simulink library "csc_pwr_power_system_sim_lib"  (R2014b)
settings: Solver=ode45  SolverMode=SingleTasking  StartTime=0.0  StopTime=10.0  RelTol=1e-3
libraries: util_info_lib x1, csc_swm_switch_state_model_collection_lib x1
settings Model: ExtModeAutoUpdateStatusClock=off  Creator=hcannon  LastModifiedBy=mstewart

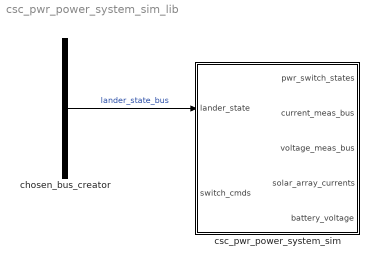
== system csc_pwr_power_system_sim_lib ==
  chosen_bus_creator : BusCreator  Inputs=7  OutDataTypeStr=Bus: lander_state_bus  NonVirtualBus=on
  csc_pwr_power_system_sim : Subsystem
  wires:
  chosen_bus_creator/1 -> csc_pwr_power_system_sim/1(lander_state)  "lander_state_bus"
  ? -> chosen_bus_creator/1  "rrd_alpha_body_in_eci"
  ? -> chosen_bus_creator/2  "rrk_rate_body_eci_body"
  ? -> chosen_bus_creator/3  "rrk_q_body_from_eci"
  ? -> chosen_bus_creator/4  "rrk_euler_zyx_rot_deg"
  ? -> chosen_bus_creator/5  "rtd_acc_body_in_eci"
  ? -> chosen_bus_creator/6  "rtk_vel_eci"
  ? -> chosen_bus_creator/7  "rtk_pos_eci"

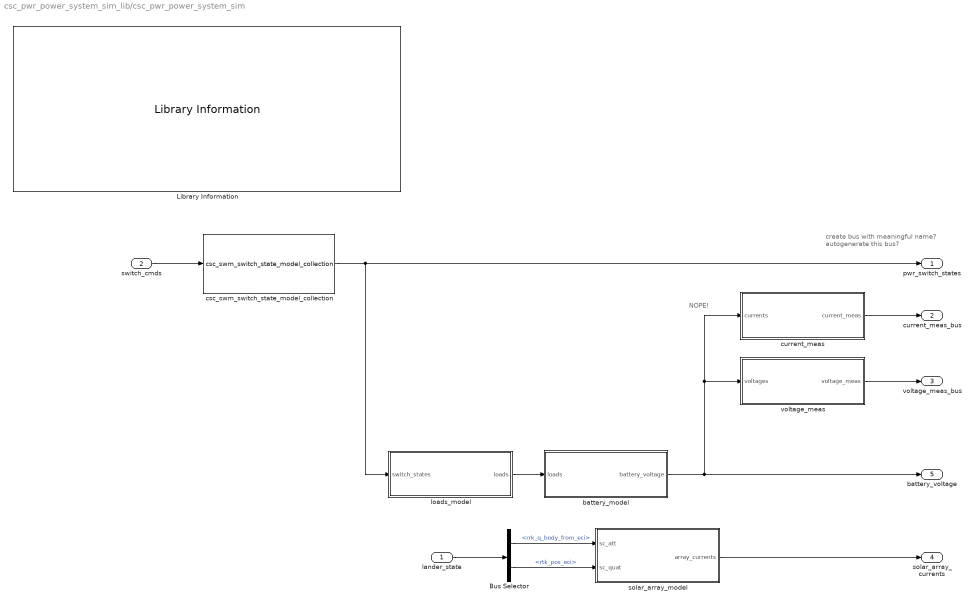
== system csc_pwr_power_system_sim_lib/csc_pwr_power_system_sim ==
  note: create bus with meaningful name?
      | autogenerate this bus?
  note: NOPE!
  lander_state : Inport
  switch_cmds : Inport  Port=2
  Bus Selector : BusSelector  OutputSignals=rrk_q_body_from_eci,rtk_pos_eci
  Library Information : util_info_lib/Library Information  owner='escrane'
  battery_model : Subsystem
  csc_swm_switch_state_model_collection : csc_swm_switch_state_model_collection_lib/csc_swm_switch_state_model_collection  SystemSampleTime=-1
  current_meas : Subsystem
  loads_model : Subsystem
  solar_array_model : Subsystem
  voltage_meas : Subsystem
  pwr_switch_states : Outport
  current_meas_bus : Outport  Port=2
  voltage_meas_bus : Outport  Port=3
  solar_array_currents : Outport  Port=4
  battery_voltage : Outport  Port=5
  wires:
  current_meas/1(current_meas) -> current_meas_bus/1
  voltage_meas/1(voltage_meas) -> voltage_meas_bus/1
  battery_model/1(battery_voltage) -> battery_voltage/1, voltage_meas/1(voltages), current_meas/1(currents)
  solar_array_model/1(array_currents) -> solar_array_currents/1
  switch_cmds/1 -> csc_swm_switch_state_model_collection/1
  loads_model/1(loads) -> battery_model/1(loads)
  csc_swm_switch_state_model_collection/1 -> loads_model/1(switch_states), pwr_switch_states/1
  Bus Selector/1 -> solar_array_model/1(sc_att)  "<rrk_q_body_from_eci>"
  Bus Selector/2 -> solar_array_model/2(sc_quat)  "<rtk_pos_eci>"
  lander_state/1 -> Bus Selector/1

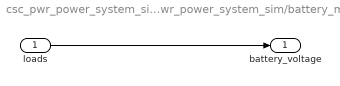
== system csc_pwr_power_system_sim_lib/csc_pwr_power_system_sim/battery_model ==
  loads : Inport
  battery_voltage : Outport
  wires:
  loads/1 -> battery_voltage/1

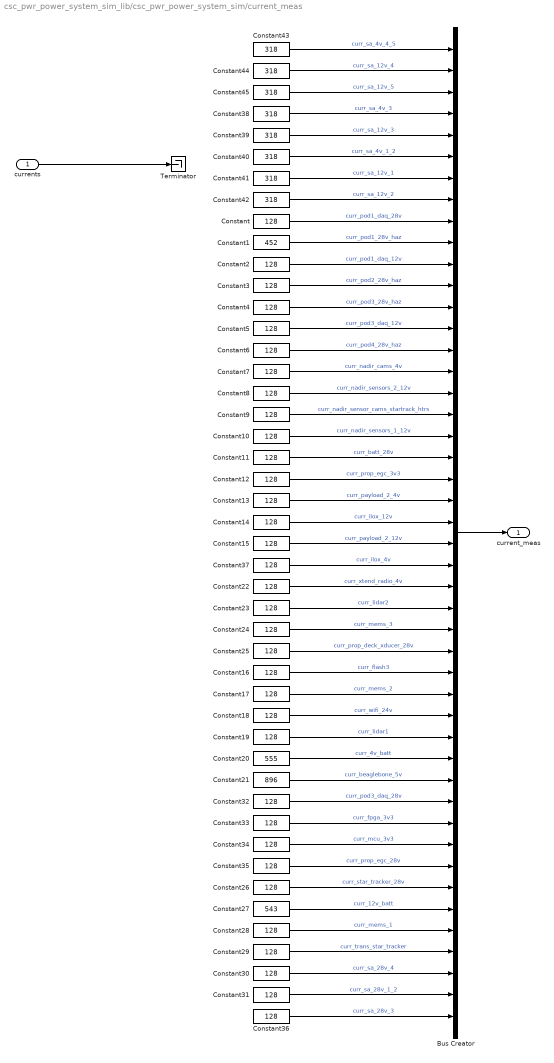
== system csc_pwr_power_system_sim_lib/csc_pwr_power_system_sim/current_meas ==
  currents : Inport
  Bus Creator : BusCreator  Inputs=46
  Constant{,2..19,22..26,28..37} (34 alike) : Constant  Value=128  OutDataTypeStr=uint16
  Constant1 : Constant  Value=452  OutDataTypeStr=uint16
  Constant20 : Constant  Value=555  OutDataTypeStr=uint16
  Constant21 : Constant  Value=896  OutDataTypeStr=uint16
  Constant27 : Constant  Value=543  OutDataTypeStr=uint16
  Constant{38..45} (8 alike) : Constant  Value=318  OutDataTypeStr=uint16
  Terminator : Terminator
  current_meas : Outport
  wires:
  Constant42/1 -> Bus Creator/8  "curr_sa_12v_2"
  Constant41/1 -> Bus Creator/7  "curr_sa_12v_1"
  Constant40/1 -> Bus Creator/6  "curr_sa_4v_1_2"
  Constant39/1 -> Bus Creator/5  "curr_sa_12v_3"
  Constant38/1 -> Bus Creator/4  "curr_sa_4v_3"
  Constant45/1 -> Bus Creator/3  "curr_sa_12v_5"
  Constant44/1 -> Bus Creator/2  "curr_sa_12v_4"
  Constant43/1 -> Bus Creator/1  "curr_sa_4v_4_5"
  Constant36/1 -> Bus Creator/46  "curr_sa_28v_3"
  Constant31/1 -> Bus Creator/45  "curr_sa_28v_1_2"
  Constant30/1 -> Bus Creator/44  "curr_sa_28v_4"
  Constant29/1 -> Bus Creator/43  "curr_trans_star_tracker"
  Constant28/1 -> Bus Creator/42  "curr_mems_1"
  Constant27/1 -> Bus Creator/41  "curr_12v_batt"
  Constant26/1 -> Bus Creator/40  "curr_star_tracker_28v"
  Constant35/1 -> Bus Creator/39  "curr_prop_egc_28v"
  Constant34/1 -> Bus Creator/38  "curr_mcu_3v3"
  Constant33/1 -> Bus Creator/37  "curr_fpga_3v3"
  Constant32/1 -> Bus Creator/36  "curr_pod3_daq_28v"
  Constant21/1 -> Bus Creator/35  "curr_beaglebone_5v"
  Constant20/1 -> Bus Creator/34  "curr_4v_batt"
  Constant19/1 -> Bus Creator/33  "curr_lidar1"
  Constant18/1 -> Bus Creator/32  "curr_wifi_24v"
  Constant17/1 -> Bus Creator/31  "curr_mems_2"
  Constant16/1 -> Bus Creator/30  "curr_flash3"
  Constant25/1 -> Bus Creator/29  "curr_prop_deck_xducer_28v"
  Constant24/1 -> Bus Creator/28  "curr_mems_3"
  Constant23/1 -> Bus Creator/27  "curr_lidar2"
  Constant22/1 -> Bus Creator/26  "curr_xtend_radio_4v"
  Constant37/1 -> Bus Creator/25  "curr_ilox_4v"
  Constant15/1 -> Bus Creator/24  "curr_payload_2_12v"
  Constant14/1 -> Bus Creator/23  "curr_ilox_12v"
  Constant13/1 -> Bus Creator/22  "curr_payload_2_4v"
  Constant12/1 -> Bus Creator/21  "curr_prop_egc_3v3"
  Constant11/1 -> Bus Creator/20  "curr_batt_28v"
  Constant10/1 -> Bus Creator/19  "curr_nadir_sensors_1_12v"
  Constant9/1 -> Bus Creator/18  "curr_nadir_sensor_cams_startrack_htrs"
  Constant8/1 -> Bus Creator/17  "curr_nadir_sensors_2_12v"
  Bus Creator/1 -> current_meas/1
  Constant7/1 -> Bus Creator/16  "curr_nadir_cams_4v"
  Constant6/1 -> Bus Creator/15  "curr_pod4_28v_haz"
  Constant5/1 -> Bus Creator/14  "curr_pod3_daq_12v"
  Constant4/1 -> Bus Creator/13  "curr_pod3_28v_haz"
  Constant3/1 -> Bus Creator/12  "curr_pod2_28v_haz"
  Constant2/1 -> Bus Creator/11  "curr_pod1_daq_12v"
  Constant1/1 -> Bus Creator/10  "curr_pod1_28v_haz"
  Constant/1 -> Bus Creator/9  "curr_pod1_daq_28v"
  currents/1 -> Terminator/1

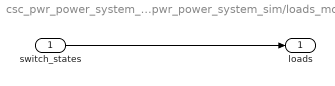
== system csc_pwr_power_system_sim_lib/csc_pwr_power_system_sim/loads_model ==
  switch_states : Inport
  loads : Outport
  wires:
  switch_states/1 -> loads/1

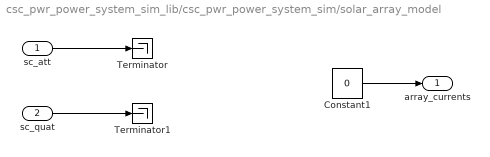
== system csc_pwr_power_system_sim_lib/csc_pwr_power_system_sim/solar_array_model ==
  sc_att : Inport
  sc_quat : Inport  Port=2
  Constant1 : Constant  Value=0  OutDataTypeStr=double
  Terminator : Terminator
  Terminator1 : Terminator
  array_currents : Outport
  wires:
  sc_att/1 -> Terminator/1
  sc_quat/1 -> Terminator1/1
  Constant1/1 -> array_currents/1

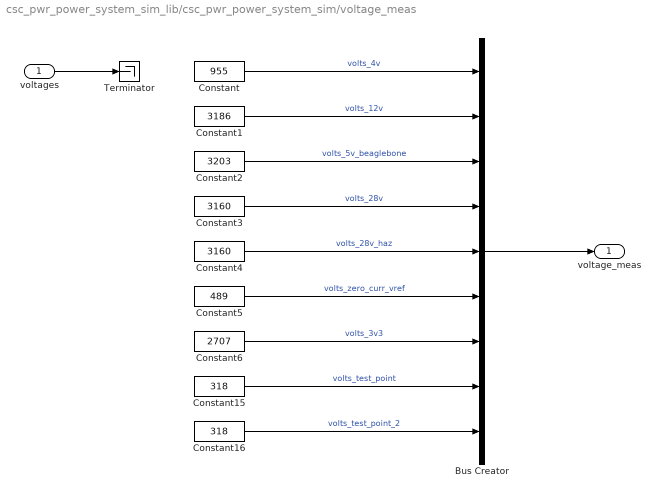
== system csc_pwr_power_system_sim_lib/csc_pwr_power_system_sim/voltage_meas ==
  voltages : Inport
  Bus Creator : BusCreator  Inputs=9
  Constant : Constant  Value=955  OutDataTypeStr=uint16
  Constant1 : Constant  Value=3186  OutDataTypeStr=uint16
  Constant15 : Constant  Value=318  OutDataTypeStr=uint16
  Constant16 : Constant  Value=318  OutDataTypeStr=uint16
  Constant2 : Constant  Value=3203  OutDataTypeStr=uint16
  Constant3 : Constant  Value=3160  OutDataTypeStr=uint16
  Constant4 : Constant  Value=3160  OutDataTypeStr=uint16
  Constant5 : Constant  Value=489  OutDataTypeStr=uint16
  Constant6 : Constant  Value=2707  OutDataTypeStr=uint16
  Terminator : Terminator
  voltage_meas : Outport
  wires:
  Constant16/1 -> Bus Creator/9  "volts_test_point_2"
  Constant15/1 -> Bus Creator/8  "volts_test_point"
  voltages/1 -> Terminator/1
  Bus Creator/1 -> voltage_meas/1
  Constant6/1 -> Bus Creator/7  "volts_3v3"
  Constant5/1 -> Bus Creator/6  "volts_zero_curr_vref"
  Constant4/1 -> Bus Creator/5  "volts_28v_haz"
  Constant3/1 -> Bus Creator/4  "volts_28v"
  Constant2/1 -> Bus Creator/3  "volts_5v_beaglebone"
  Constant1/1 -> Bus Creator/2  "volts_12v"
  Constant/1 -> Bus Creator/1  "volts_4v"
